simulink model "Q8_b"  (R2021b)
settings: Solver=VariableStepAuto  StartTime=0.0  StopTime=10.0  RelTol=1e-3
undefined symbols (not defined in the file): A_numerical, B_numerical, B_parameter, C_numerical, D_numerical, g
settings Model: Creator=sadeg  LastModifiedBy=sadeg

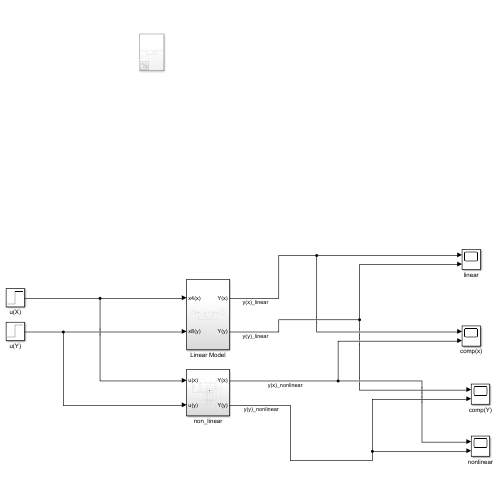
[thumbnail: Simulink's stored preview of the top-level diagram]
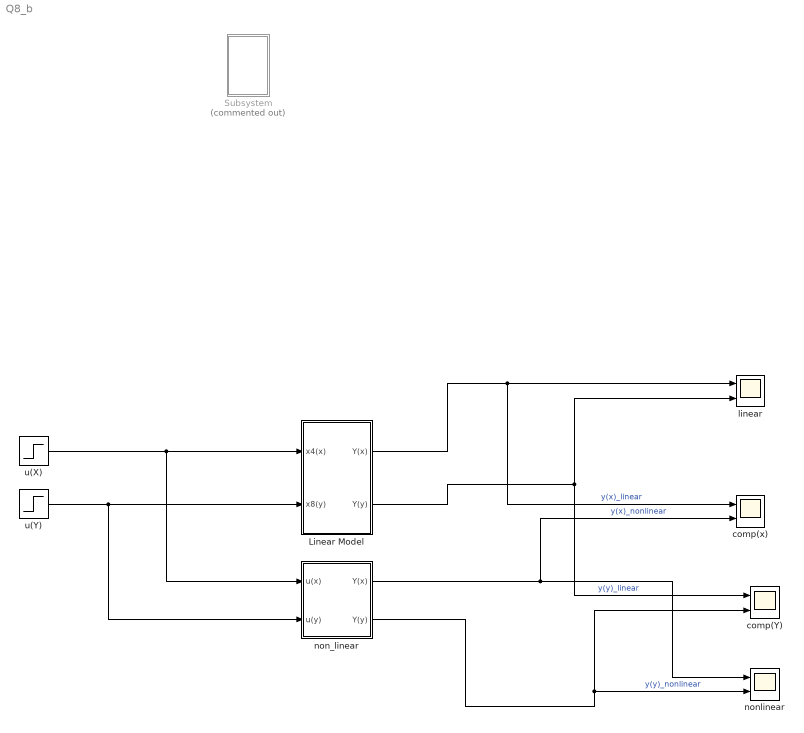
== system Q8_b ==
  Linear Model : Subsystem
  Subsystem : Subsystem  Commented=on
  comp(Y) : Scope  NumInputPorts=2
  comp(x) : Scope  NumInputPorts=2
  linear : Scope  NumInputPorts=2
  non_linear : Subsystem
  nonlinear : Scope  NumInputPorts=2
  u(X) : Step  After=0.1  SampleTime=0
  u(Y) : Step  After=0.1  SampleTime=0
  wires:
  Linear Model/1(Y(x)) -> comp(x)/1, linear/1  "y(x)_linear"
  Linear Model/2(Y(y)) -> comp(Y)/1, linear/2  "y(y)_linear"
  u(X)/1 -> non_linear/1(u(x)), Linear Model/1(x4(x))
  u(Y)/1 -> non_linear/2(u(y)), Linear Model/2(x8(y))
  non_linear/1(Y(x)) -> nonlinear/1, comp(x)/2  "y(x)_nonlinear"
  non_linear/2(Y(y)) -> nonlinear/2, comp(Y)/2  "y(y)_nonlinear"

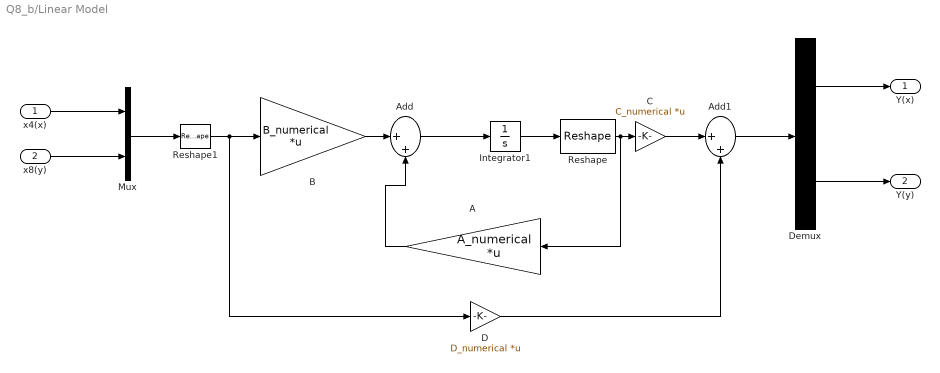
== system Q8_b/Linear Model ==
  x4(x) : Inport
  x8(y) : Inport  Port=2
  A : Gain  Gain=A_numerical  Multiplication=Matrix(K*u)
  Add : Sum  Inputs=|++
  Add1 : Sum  Inputs=|++
  B : Gain  Gain=B_numerical  Multiplication=Matrix(K*u)
  C : Gain  Gain=C_numerical  Multiplication=Matrix(K*u)
  D : Gain  Gain=D_numerical  Multiplication=Matrix(K*u)
  Demux : Demux  Outputs=2
  Integrator1 : Integrator  InitialCondition=zeros(8,1)
  Mux : Mux  Inputs=2
  Reshape : Reshape  OutputDimensionality=Column vector (2-D)
  Reshape1 : Reshape  OutputDimensionality=Column vector (2-D)
  Y(x) : Outport
  Y(y) : Outport  Port=2
  wires:
  Demux/2 -> Y(y)/1
  A/1 -> Add/2
  Integrator1/1 -> Reshape/1
  Reshape/1 -> A/1, C/1
  x4(x)/1 -> Mux/1
  C/1 -> Add1/1
  B/1 -> Add/1
  x8(y)/1 -> Mux/2
  Demux/1 -> Y(x)/1
  Add1/1 -> Demux/1
  Add/1 -> Integrator1/1
  Reshape1/1 -> D/1, B/1
  Mux/1 -> Reshape1/1
  D/1 -> Add1/2

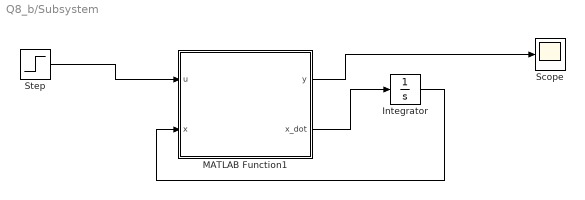
== system Q8_b/Subsystem ==
  Integrator : Integrator  InitialCondition=zeros(8,1)
  MATLAB Function1 : MATLAB Function  TreatAsAtomicUnit=on
  Scope : Scope
  Step : Step  SampleTime=0
  wires:
  Integrator/1 -> MATLAB Function1/2(x)
  MATLAB Function1/1(y) -> Scope/1
  Step/1 -> MATLAB Function1/1(u)
  MATLAB Function1/2(x_dot) -> Integrator/1

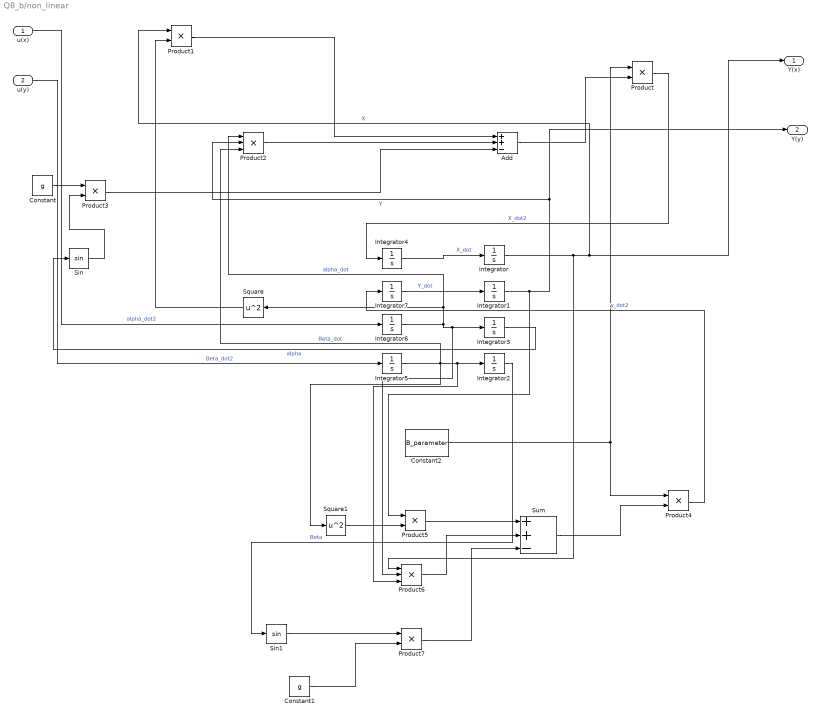
== system Q8_b/non_linear ==
  u(x) : Inport
  u(y) : Inport  Port=2
  Add : Sum  Inputs=++-
  Constant : Constant  Value=g
  Constant1 : Constant  Value=g
  Constant2 : Constant  Value=B_parameter
  Integrator{,1..7} (8 alike) : Integrator
  Product{,1,3..5,7} (6 alike) : Product
  Product2 : Product  Inputs=3
  Product6 : Product  Inputs=3
  Sin : Trigonometry
  Sin1 : Trigonometry
  Square : Math  Operator=square  SaturateOnIntegerOverflow=on
  Square1 : Math  Operator=square  SaturateOnIntegerOverflow=on
  Sum : Sum  Inputs=++-
  Y(x) : Outport
  Y(y) : Outport  Port=2
  wires:
  Constant2/1 -> Product/1, Product4/1
  Add/1 -> Product/2
  Product1/1 -> Add/1
  Product2/1 -> Add/2
  Product3/1 -> Add/3
  Integrator/1 -> Product6/1, Y(x)/1, Product1/1  "X"
  Integrator4/1 -> Integrator/1  "X_dot"
  Integrator7/1 -> Integrator1/1  "Y_dot"
  Integrator1/1 -> Product5/1, Y(y)/1, Product2/2  "Y"
  Integrator5/1 -> Square1/1, Product2/3, Product6/3, Integrator2/1  "Beta_dot"
  Integrator2/1 -> Sin1/1  "Beta"
  Square/1 -> Product1/2
  Integrator3/1 -> Sin/1  "alpha"
  Integrator6/1 -> Product6/2, Integrator3/1, Product2/1, Square/1  "alpha_dot"
  u(x)/1 -> Integrator6/1  "alpha_dot2"
  Product4/1 -> Integrator7/1  "y_dot2"
  Product/1 -> Integrator4/1  "X_dot2"
  u(y)/1 -> Integrator5/1  "Beta_dot2"
  Constant/1 -> Product3/1
  Sin/1 -> Product3/2
  Sum/1 -> Product4/2
  Product5/1 -> Sum/1
  Product7/1 -> Sum/3
  Product6/1 -> Sum/2
  Sin1/1 -> Product7/1
  Constant1/1 -> Product7/2
  Square1/1 -> Product5/2

== matlab function Q8_b/Subsystem/MATLAB Function1 ==
  data: u input size=2; x input size=8; y output size=2; x_dot output size=8; A_numerical parameter size=8x8; B_numerical parameter size=8x2; C_numerical parameter size=2x8; D_numerical parameter size=2x2
% function [y,x_dot] = fcn(u, x ,A_numerical, B_numerical, C_numerical)
% % A1 = [x(2),B_parameter*(x(1)*x(4)^2 + x(4)*x(5)*x(8) -g*sin(x(3))),x(4),0];
% % A2 = [x(6),B_parameter*(x(5)*x(8)^2 + x(1)*x(4)*x(8) -g*sin(x(7))),x(8),0];
% % A = [A1,A2]';
% % B = [0,0;0,0;0,0;1,0;0,0;0,0;0,0;0,1];
% % C = [1,0,0,0,0,0,0,0;0,0,0,0,1,0,0,0];
% % D = [0;0];
% % x_balance = [0,0,0,0,0,0,0,0];
% % A_linear = jacobian(A,x);
% % A_numerical = double(subs(A_linear,[x1,x1_dot,a1,a1_dot,y1,y1_dot,b1,b1_dot],[0,0,0,0,0,0,0,0]));
% % B_numerical = B;
% % C_numerical = C;
% % D_numerical = D;
% % 
% 
% 
% 
% 
% 
% 
% x_dot = A_numerical*x + B_numerical*u;
% y = C_numerical*x ;
% 
% function [y, x_dot] = fcn(u, x, A_numerical, B_numerical, C_numerical, D_numerical)
%     % Predefine output sizes
%     x_dot = zeros(8, 1); % 8x1 state derivative
%     y = zeros(2, 1);     % 2x1 output
% 
%     % Compute state derivatives and outputs
%     x_dot = A_numerical * x + B_numerical * u;
%     y = C_numerical * x + D_numerical * u;
function [y, x_dot] = fcn(u, x, A_numerical, B_numerical, C_numerical, D_numerical)
    % Predefine output sizes
    x_dot = zeros(8, 1); % 8x1 state derivative
    y = zeros(2, 1);     % 2x1 output

    % Check dimensions for safety (optional for debugging)
    assert(isequal(size(A_numerical), [8, 8]), 'A_numerical must be 8x8');
    assert(isequal(size(B_numerical), [8, 2]), 'B_numerical must be 8x2');
    assert(isequal(size(C_numerical), [2, 8]), 'C_numerical must be 2x8');
    assert(isequal(size(D_numerical), [2, 2]), 'D_numerical must be 2x2');
    assert(isequal(size(x), [8, 1]), 'x must be 8x1');
    assert(isequal(size(u), [2, 1]), 'u must be 2x1');

    % Compute state derivatives and outputs
    x_dot = A_numerical * x + B_numerical * u;
    y = C_numerical * x + D_numerical * u;
end
